simulink model "traffic_cop_eyes"  (Simulink 8.7)
settings: Solver=FixedStepAuto  StartTime=0.0  StopTime=10.0  FixedStep=0.01  RelTol=1e-3
settings Model: Creator=eispin  LastModifiedBy=eispin
settings DataIOCC: LimitDataPoints=off  SaveFormat=Dataset
settings DebuggingCC: UnderspecifiedInitializationDetection=Simplified  MergeDetectMultiDrivingBlocksExec=error
settings HardwareCC: ProdBitPerPointer=64  ProdLargestAtomicFloat=Float  ProdIntDivRoundTo=Zero  ProdEndianess=LittleEndian  ProdWordSize=64  ProdHWDeviceType=Intel->x86-64 (Windows64)
settings ModelReferenceCC: PropagateSignalLabelsOutOfModel=on
settings ConfigComp: CovModelRefEnable=off

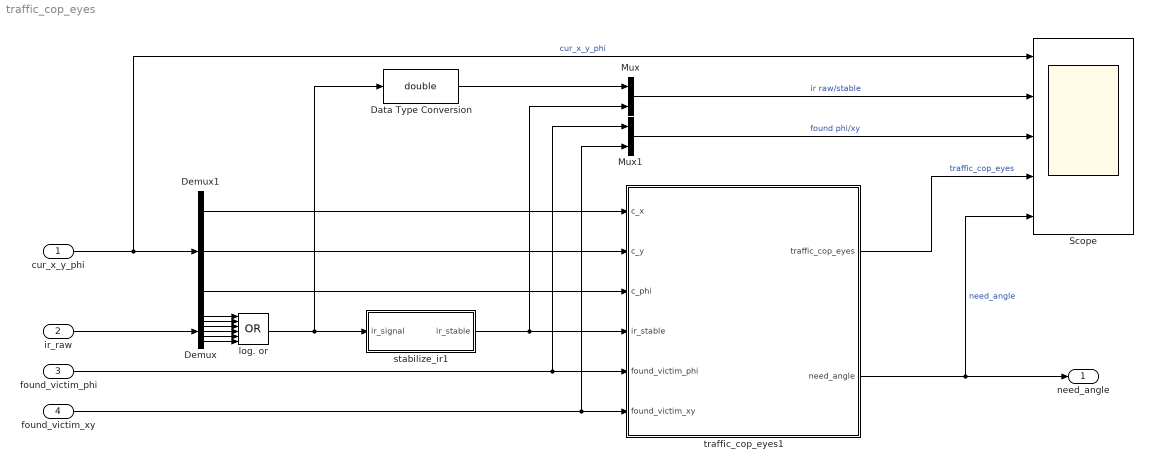
== system traffic_cop_eyes ==
  cur_x_y_phi : Inport
  ir_raw : Inport  Port=2
  found_victim_phi : Inport  Port=3
  found_victim_xy : Inport  Port=4
  Data Type Conversion : DataTypeConversion  OutDataTypeStr=double
  Demux : Demux  Outputs=6
  Demux1 : Demux  Outputs=3
  Mux : Mux  Inputs=2
  Mux1 : Mux  Inputs=2
  Scope : Scope  NumInputPorts=5
  log. or : Logic  Operator=OR  Inputs=6  AllPortsSameDT=off  OutDataTypeStr=boolean
  stabilize_ir1 : Stateflow chart  TreatAsAtomicUnit=on
  traffic_cop_eyes1 : Stateflow chart  TreatAsAtomicUnit=on
  need_angle : Outport
  wires:
  found_victim_xy/1 -> traffic_cop_eyes1/6(found_victim_xy), Mux1/2
  log. or/1 -> Data Type Conversion/1, stabilize_ir1/1(ir_signal)
  Demux/3 -> log. or/3
  Demux/2 -> log. or/2
  traffic_cop_eyes1/2(need_angle) -> need_angle/1, Scope/5  "need_angle"
  stabilize_ir1/1(ir_stable) -> traffic_cop_eyes1/4(ir_stable), Mux/2
  found_victim_phi/1 -> traffic_cop_eyes1/5(found_victim_phi), Mux1/1
  Demux/6 -> log. or/6
  Demux/5 -> log. or/5
  cur_x_y_phi/1 -> Scope/1, Demux1/1  "cur_x_y_phi"
  Demux/1 -> log. or/1
  Demux/4 -> log. or/4
  Demux1/2 -> traffic_cop_eyes1/2(c_y)
  Demux1/1 -> traffic_cop_eyes1/1(c_x)
  ir_raw/1 -> Demux/1
  traffic_cop_eyes1/1(traffic_cop_eyes) -> Scope/4  "traffic_cop_eyes"
  Demux1/3 -> traffic_cop_eyes1/3(c_phi)
  Mux/1 -> Scope/2  "ir raw/stable"
  Mux1/1 -> Scope/3  "found phi/xy"
  Data Type Conversion/1 -> Mux/1

== stateflow chart traffic_cop_eyes1 ==
  state Detection
    state WaitDetect
      en:
      last_x = c_x;
      last_y = c_y;
      last_phi = c_phi;
      need_angle = 1;
      ex:
      need_angle = 0;
    state NoIdea
    state WaitOff
    state SomeIdea
    (default) -> NoIdea
    NoIdea -> WaitDetect : [ir_stable == 1]
    SomeIdea -> WaitDetect : [ir_stable == 1 && ...
        |  ray_dist(c_x-last_x, c_y-last_y, last_phi) >= min_dist]
    WaitDetect -> WaitOff : [found_victim_phi == 1]
    WaitOff -> SomeIdea : [found_victim_phi == 0]
  state Done
    en:
    need_angle = 0;
  (default) -> Detection
  Detection -> Done : [found_victim_xy == 1]
  data: dx function_input double; dy function_input double; ray_phi function_input double; dist function_output double; traffic_cop_eyes output Enum: traffic_cop_eyesModeType; c_x input double; c_y input double; c_phi input double; ir_stable input double; found_victim_phi input double; found_victim_xy input double; last_x local double; last_y local double; min_dist constant double =13; need_angle output double; last_phi local double
  function dist = ray_dist(dx, dy, ray_phi):
    | function dist = ray_dist(dx, dy, ray_phi)
    | 
    | dv = [dx dy];
    | %ray_v = [cos(ray_phi) sin(ray_phi)];
    | ray_v_orth = [-sin(ray_phi); cos(ray_phi)];
    | dist = abs(dv * ray_v_orth);
    | 
    | end

== stateflow chart stabilize_ir1 ==
  state Nothing
  state Teddy
    en:
    ir_stable = 1;
    ex:
    ir_stable = 0;
  state Something
  (default) -> Nothing
  Teddy -> Nothing : [ir_signal == 0]
  Something -> Nothing [order 1] : [ir_signal == 0]
  Nothing -> Something : [ir_signal == 1]
  Something -> Teddy [order 2] : [after(1,sec)]
  data: ir_signal input double; ir_stable output double
